simulink model "CF010A_GmTqArbn"  (R2013b)
settings: Solver=FixedStepDiscrete  SolverMode=SingleTasking  StartTime=0.0  StopTime=1  FixedStep=0.002  RelTol=1e-3
values from neighbouring files (symbols this model uses):
  ARCHGLBPRM_2MILLISEC_SEC_F32 = DataDict.Constant    [CF010A_GmTqArbn_DataDict.m]
  ESCCMDACTV_CNT_U08 = DataDict.Constant    [CF010A_GmTqArbn_DataDict.m]
  ESCCMDTMPLIMD_CNT_U08 = DataDict.Constant    [CF010A_GmTqArbn_DataDict.m]
  ESCTQCMDOVRLLIM_HWNWTMTR_F32 = DataDict.Constant    [CF010A_GmTqArbn_DataDict.m]
  FINALSLEWLWRLIM_HWNWTMTRPERSEC_F32 = DataDict.Constant    [CF010A_GmTqArbn_DataDict.m]
  GmTqArbnApaAssiScaEna = DataDict.Calibration    [CF010A_GmTqArbn_DataDict.m]
  GmTqArbnApaDampgScaEna = DataDict.Calibration    [CF010A_GmTqArbn_DataDict.m]
  GmTqArbnApaEnaRate = DataDict.Calibration    [CF010A_GmTqArbn_DataDict.m]
  GmTqArbnApaRtnScaEna = DataDict.Calibration    [CF010A_GmTqArbn_DataDict.m]
  GmTqArbnEscMaxTq = DataDict.Calibration    [CF010A_GmTqArbn_DataDict.m]
  GmTqArbnLkaSlewEna = DataDict.Calibration    [CF010A_GmTqArbn_DataDict.m]
  HWTQCMDOVRLLIM_HWNWTMTR_F32 = DataDict.Constant    [CF010A_GmTqArbn_DataDict.m]
  LKACMDHILIM_HWNWTMTR_F32 = DataDict.Constant    [CF010A_GmTqArbn_DataDict.m]
  LKASTACTV_CNT_U08 = DataDict.Constant    [CF010A_GmTqArbn_DataDict.m]
  LKATQCMDOVRLLIM_HWNWTMTR_F32 = DataDict.Constant    [CF010A_GmTqArbn_DataDict.m]
  MOTTQCMDOVRLLIM_MOTNWTMTR_F32 = DataDict.Constant    [CF010A_GmTqArbn_DataDict.m]
  OUTPCMDHILIM_ULS_F32 = DataDict.Constant    [CF010A_GmTqArbn_DataDict.m]
  OUTPCMDLOWRLIM_ULS_F32 = DataDict.Constant    [CF010A_GmTqArbn_DataDict.m]
  POSNSERVOSMOOTHMINLWRLIM_ULSPERSEC_F32 = DataDict.Constant    [CF010A_GmTqArbn_DataDict.m]
  VELDPTTQOVRLMTRCOFFS_HWNWTMTRPERSEC_F32 = DataDict.Constant    [CF010A_GmTqArbn_DataDict.m]
  VELDPTTQOVRLMTRCTQPERVEHSPD_HWNWTMTRPERSECPERKPH_F32 = DataDict.Constant    [CF010A_GmTqArbn_DataDict.m]
libraries: NxtrLim x11, NexteerUtilities x8, FixdToFloat x3, Fil x2, NxtrAbslt x2, simulink x2
(part 4 of 4)

== system CF010A_GmTqArbn/GmTqArbn/GmTqArbnPer1/ESC logic/THEN7 ==
  note: Change Log:
      | Oct 12, 2012  Created by Kevin Derry as a 1-input, 1-output block
      | Nov 30, 2012  dynamically configurable for 1 to 5 ports.
  note: Do not modify these blocks manually.  They
      | are generated programatically.  Changing the
      | number of blocks available or their names requires
      | corresponding changes to Callback and Initialization
      | routines.
      |
      | Do not change the "Display" tab of mask editor.  The
      | outport names are created programatically in the
      | "Initialize" section.
  In1 : Inport
  Action Port : ActionPort  ActionType=then
  In{2..5} (4 alike) : Ground
  Out{2..5} (4 alike) : Terminator
  Out1 : Outport
  wires:
  In1/1 -> Out1/1
  In2/1 -> Out2/1
  In3/1 -> Out3/1
  In4/1 -> Out4/1
  In5/1 -> Out5/1

== system CF010A_GmTqArbn/GmTqArbn/GmTqArbnPer1/ESC logic/THEN8 ==
  note: Do not modify these blocks manually.  They
      | are generated programatically.  Changing the
      | number of blocks available or their names requires
      | corresponding changes to Callback and Initialization
      | routines.
      |
      | Do not change the "Display" tab of mask editor.  The
      | outport names are created programatically in the
      | "Initialize" section.
  note: Change Log:
      | Oct 12, 2012  Created by Kevin Derry as a 1-input, 1-output block
      | Nov 30, 2012  dynamically configurable for 1 to 5 ports.
  In1 : Inport
  Action Port : ActionPort  ActionType=else
  In{2..5} (4 alike) : Ground
  Out{2..5} (4 alike) : Terminator
  Out1 : Outport
  wires:
  In5/1 -> Out5/1
  In4/1 -> Out4/1
  In3/1 -> Out3/1
  In2/1 -> Out2/1
  In1/1 -> Out1/1

== system CF010A_GmTqArbn/GmTqArbn/GmTqArbnPer1/PosnServo_Smoothed_Ramp/CopyRight2 ==

== system CF010A_GmTqArbn/GmTqArbn/GmTqArbnPer1/PosnServo_Smoothed_Ramp/THEN1 ==
  note: Do not modify these blocks manually.  They
      | are generated programatically.  Changing the
      | number of blocks available or their names requires
      | corresponding changes to Callback and Initialization
      | routines.
      |
      | Do not change the "Display" tab of mask editor.  The
      | outport names are created programatically in the
      | "Initialize" section.
  note: Change Log:
      | Oct 12, 2012  Created by Kevin Derry as a 1-input, 1-output block
      | Nov 30, 2012  dynamically configurable for 1 to 5 ports.
  In1 : Inport
  Action Port : ActionPort  ActionType=then
  In{2..5} (4 alike) : Ground
  Out{2..5} (4 alike) : Terminator
  Out1 : Outport
  wires:
  In5/1 -> Out5/1
  In4/1 -> Out4/1
  In3/1 -> Out3/1
  In2/1 -> Out2/1
  In1/1 -> Out1/1

== system CF010A_GmTqArbn/GmTqArbn/GmTqArbnPer1/PosnServo_Smoothed_Ramp/THEN2 ==
  note: Change Log:
      | Oct 12, 2012  Created by Kevin Derry as a 1-input, 1-output block
      | Nov 30, 2012  dynamically configurable for 1 to 5 ports.
  note: Do not modify these blocks manually.  They
      | are generated programatically.  Changing the
      | number of blocks available or their names requires
      | corresponding changes to Callback and Initialization
      | routines.
      |
      | Do not change the "Display" tab of mask editor.  The
      | outport names are created programatically in the
      | "Initialize" section.
  In1 : Inport
  Action Port : ActionPort  ActionType=else
  In{2..5} (4 alike) : Ground
  Out{2..5} (4 alike) : Terminator
  Out1 : Outport
  wires:
  In1/1 -> Out1/1
  In2/1 -> Out2/1
  In3/1 -> Out3/1
  In4/1 -> Out4/1
  In5/1 -> Out5/1

== system CF010A_GmTqArbn/GmTqArbn/GmTqArbnPer1/PosnServo_Smoothed_Ramp/THEN3 ==
  note: Change Log:
      | Oct 12, 2012  Created by Kevin Derry as a 1-input, 1-output block
      | Nov 30, 2012  dynamically configurable for 1 to 5 ports.
  note: Do not modify these blocks manually.  They
      | are generated programatically.  Changing the
      | number of blocks available or their names requires
      | corresponding changes to Callback and Initialization
      | routines.
      |
      | Do not change the "Display" tab of mask editor.  The
      | outport names are created programatically in the
      | "Initialize" section.
  In1 : Inport
  Action Port : ActionPort  ActionType=then
  In{2..5} (4 alike) : Ground
  Out{2..5} (4 alike) : Terminator
  Out1 : Outport
  wires:
  In1/1 -> Out1/1
  In2/1 -> Out2/1
  In3/1 -> Out3/1
  In4/1 -> Out4/1
  In5/1 -> Out5/1

== system CF010A_GmTqArbn/GmTqArbn/GmTqArbnPer1/PosnServo_Smoothed_Ramp/THEN4 ==
  note: Do not modify these blocks manually.  They
      | are generated programatically.  Changing the
      | number of blocks available or their names requires
      | corresponding changes to Callback and Initialization
      | routines.
      |
      | Do not change the "Display" tab of mask editor.  The
      | outport names are created programatically in the
      | "Initialize" section.
  note: Change Log:
      | Oct 12, 2012  Created by Kevin Derry as a 1-input, 1-output block
      | Nov 30, 2012  dynamically configurable for 1 to 5 ports.
  In1 : Inport
  Action Port : ActionPort  ActionType=else
  In{2..5} (4 alike) : Ground
  Out{2..5} (4 alike) : Terminator
  Out1 : Outport
  wires:
  In5/1 -> Out5/1
  In4/1 -> Out4/1
  In3/1 -> Out3/1
  In2/1 -> Out2/1
  In1/1 -> Out1/1

== system CF010A_GmTqArbn/GmTqArbn/GmTqArbnPer1/PosnServo_Smoothed_Ramp/THEN5 ==
  note: Change Log:
      | Oct 12, 2012  Created by Kevin Derry as a 1-input, 1-output block
      | Nov 30, 2012  dynamically configurable for 1 to 5 ports.
  note: Do not modify these blocks manually.  They
      | are generated programatically.  Changing the
      | number of blocks available or their names requires
      | corresponding changes to Callback and Initialization
      | routines.
      |
      | Do not change the "Display" tab of mask editor.  The
      | outport names are created programatically in the
      | "Initialize" section.
  In1 : Inport
  Action Port : ActionPort  ActionType=then
  In{2..5} (4 alike) : Ground
  Out{2..5} (4 alike) : Terminator
  Out1 : Outport
  wires:
  In1/1 -> Out1/1
  In2/1 -> Out2/1
  In3/1 -> Out3/1
  In4/1 -> Out4/1
  In5/1 -> Out5/1

== system CF010A_GmTqArbn/GmTqArbn/GmTqArbnPer1/PosnServo_Smoothed_Ramp/THEN6 ==
  note: Do not modify these blocks manually.  They
      | are generated programatically.  Changing the
      | number of blocks available or their names requires
      | corresponding changes to Callback and Initialization
      | routines.
      |
      | Do not change the "Display" tab of mask editor.  The
      | outport names are created programatically in the
      | "Initialize" section.
  note: Change Log:
      | Oct 12, 2012  Created by Kevin Derry as a 1-input, 1-output block
      | Nov 30, 2012  dynamically configurable for 1 to 5 ports.
  In1 : Inport
  Action Port : ActionPort  ActionType=else
  In{2..5} (4 alike) : Ground
  Out{2..5} (4 alike) : Terminator
  Out1 : Outport
  wires:
  In5/1 -> Out5/1
  In4/1 -> Out4/1
  In3/1 -> Out3/1
  In2/1 -> Out2/1
  In1/1 -> Out1/1

== system CF010A_GmTqArbn/GmTqArbn/GmTqArbnPer1/Ramp to Value/CopyRight2 ==

== system CF010A_GmTqArbn/GmTqArbn/GmTqArbnPer1/Ramp to Value/THEN1 ==
  note: Do not modify these blocks manually.  They
      | are generated programatically.  Changing the
      | number of blocks available or their names requires
      | corresponding changes to Callback and Initialization
      | routines.
      |
      | Do not change the "Display" tab of mask editor.  The
      | outport names are created programatically in the
      | "Initialize" section.
  note: Change Log:
      | Oct 12, 2012  Created by Kevin Derry as a 1-input, 1-output block
      | Nov 30, 2012  dynamically configurable for 1 to 5 ports.
  In1 : Inport
  Action Port : ActionPort  ActionType=then
  In{2..5} (4 alike) : Ground
  Out{2..5} (4 alike) : Terminator
  Out1 : Outport
  wires:
  In5/1 -> Out5/1
  In4/1 -> Out4/1
  In3/1 -> Out3/1
  In2/1 -> Out2/1
  In1/1 -> Out1/1

== system CF010A_GmTqArbn/GmTqArbn/GmTqArbnPer1/Ramp to Value/THEN2 ==
  note: Change Log:
      | Oct 12, 2012  Created by Kevin Derry as a 1-input, 1-output block
      | Nov 30, 2012  dynamically configurable for 1 to 5 ports.
  note: Do not modify these blocks manually.  They
      | are generated programatically.  Changing the
      | number of blocks available or their names requires
      | corresponding changes to Callback and Initialization
      | routines.
      |
      | Do not change the "Display" tab of mask editor.  The
      | outport names are created programatically in the
      | "Initialize" section.
  In1 : Inport
  Action Port : ActionPort  ActionType=else
  In{2..5} (4 alike) : Ground
  Out{2..5} (4 alike) : Terminator
  Out1 : Outport
  wires:
  In1/1 -> Out1/1
  In2/1 -> Out2/1
  In3/1 -> Out3/1
  In4/1 -> Out4/1
  In5/1 -> Out5/1

== system CF010A_GmTqArbn/GmTqArbn/GmTqArbnPer1/Ramp to Value/THEN3 ==
  note: Change Log:
      | Oct 12, 2012  Created by Kevin Derry as a 1-input, 1-output block
      | Nov 30, 2012  dynamically configurable for 1 to 5 ports.
  note: Do not modify these blocks manually.  They
      | are generated programatically.  Changing the
      | number of blocks available or their names requires
      | corresponding changes to Callback and Initialization
      | routines.
      |
      | Do not change the "Display" tab of mask editor.  The
      | outport names are created programatically in the
      | "Initialize" section.
  In1 : Inport
  Action Port : ActionPort  ActionType=then
  In{2..5} (4 alike) : Ground
  Out{2..5} (4 alike) : Terminator
  Out1 : Outport
  wires:
  In1/1 -> Out1/1
  In2/1 -> Out2/1
  In3/1 -> Out3/1
  In4/1 -> Out4/1
  In5/1 -> Out5/1

== system CF010A_GmTqArbn/GmTqArbn/GmTqArbnPer1/Ramp to Value/THEN4 ==
  note: Do not modify these blocks manually.  They
      | are generated programatically.  Changing the
      | number of blocks available or their names requires
      | corresponding changes to Callback and Initialization
      | routines.
      |
      | Do not change the "Display" tab of mask editor.  The
      | outport names are created programatically in the
      | "Initialize" section.
  note: Change Log:
      | Oct 12, 2012  Created by Kevin Derry as a 1-input, 1-output block
      | Nov 30, 2012  dynamically configurable for 1 to 5 ports.
  In1 : Inport
  Action Port : ActionPort  ActionType=else
  In{2..5} (4 alike) : Ground
  Out{2..5} (4 alike) : Terminator
  Out1 : Outport
  wires:
  In5/1 -> Out5/1
  In4/1 -> Out4/1
  In3/1 -> Out3/1
  In2/1 -> Out2/1
  In1/1 -> Out1/1
